simulink model "slb_complex_mult"  (R2015b)
settings: Solver=FixedStepDiscrete  SolverMode=SingleTasking  StartTime=0.0  StopTime=10  RelTol=1e-3
settings Model: DataTypeOverride=Off  Creator=amatsumo  LastModifiedBy=amatsumo
settings DataIOCC: SaveFormat=Array  SaveOutput=off  SignalLogging=off  SaveTime=off
settings OptimizationCC: BlockReduction=off  ConditionallyExecuteInputs=off  DefaultParameterBehavior=Inlined
settings DebuggingCC: AlgebraicLoopMsg=error  UnderspecifiedInitializationDetection=Classic  MergeDetectMultiDrivingBlocksExec=none  SolverPrmCheckMsg=warning  SingleTaskRateTransMsg=error  StateNameClashWarn=warning
settings HardwareCC: ProdBitPerPointer=32  ProdLargestAtomicFloat=None  ProdIntDivRoundTo=Undefined  ProdEndianess=Unspecified  ProdWordSize=32  ProdHWDeviceType=ASIC/FPGA->ASIC/FPGA  ProdEqTarget=off
settings GRTTargetCC: GeneratePreprocessorConditionals=Disable all
settings ConfigComp: CovModelRefEnable=Off  CovSFcnEnable=off

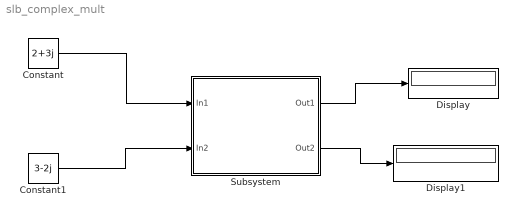
== system slb_complex_mult ==
  Constant : Constant  Value=2+3j  OutDataTypeStr=fixdt(1,16,12)  SampleTime=1
  Constant1 : Constant  Value=3-2j  OutDataTypeStr=fixdt(1,16,12)  SampleTime=1
  Display : Display
  Display1 : Display
  Subsystem : Subsystem
  wires:
  Constant/1 -> Subsystem/1(In1)
  Constant1/1 -> Subsystem/2(In2)
  Subsystem/1(Out1) -> Display/1
  Subsystem/2(Out2) -> Display1/1

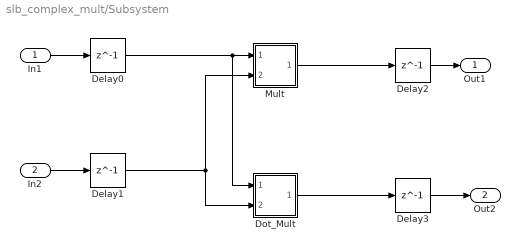
== system slb_complex_mult/Subsystem ==
  In1 : Inport
  In2 : Inport  Port=2
  Delay{0..3} (4 alike) : Delay  DelayLength=1
  Dot_Mult : Subsystem
  Mult : Subsystem
  Out1 : Outport
  Out2 : Outport  Port=2
  wires:
  In1/1 -> Delay0/1
  In2/1 -> Delay1/1
  Delay3/1 -> Out2/1
  Delay2/1 -> Out1/1
  Delay0/1 -> Dot_Mult/1(In1), Mult/1(In1)
  Mult/1(Out1) -> Delay2/1
  Dot_Mult/1(Out1) -> Delay3/1
  Delay1/1 -> Dot_Mult/2(In2), Mult/2(In2)

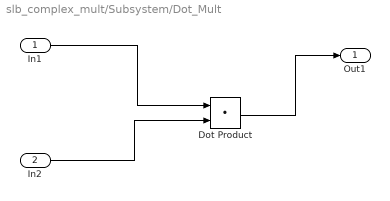
== system slb_complex_mult/Subsystem/Dot_Mult ==
  In1 : Inport
  In2 : Inport  Port=2
  Dot Product : DotProduct  InputSameDT=on  OutDataTypeStr=Inherit: Inherit via internal rule
  Out1 : Outport
  wires:
  In1/1 -> Dot Product/1
  Dot Product/1 -> Out1/1
  In2/1 -> Dot Product/2

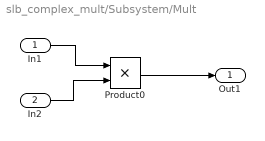
== system slb_complex_mult/Subsystem/Mult ==
  In1 : Inport
  In2 : Inport  Port=2
  Product0 : Product
  Out1 : Outport
  wires:
  In2/1 -> Product0/2
  Product0/1 -> Out1/1
  In1/1 -> Product0/1
